simulink model "exercicio3"  (R2018b)
settings: Solver=VariableStepAuto  StartTime=0.0  StopTime=10.0  RelTol=1e-3
values from neighbouring files (symbols this model uses):
  A = [   -1,    1,    2,    2.5 ... (first row only)    [exercicio_01.m]    (also in exercicio_03.m = [-2.068, -2; 2, 0]; exercicio_03_2.m = [-2.068, -2; 2, 0])
  B = [1; 0]    [exercicio_03.m]    (also in exercicio_03_2.m)
  C = [1, -0.4]    [exercicio_03.m]    (also in exercicio_03_2.m)
  D = 0    [exercicio_03.m]    (also in exercicio_03_2.m)
settings Model: Creator=bernardo  LastModifiedBy=bernardo

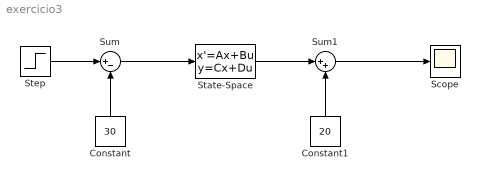
== system exercicio3 ==
  Constant : Constant  Value=30
  Constant1 : Constant  Value=20
  Scope : Scope
  State-Space : StateSpace  A=A  B=B  C=C  D=D  InitialCondition=0.1
  Step : Step  Time=0  After=25  SampleTime=0.001
  Sum : Sum  Inputs=|+-
  Sum1 : Sum  Inputs=|++
  wires:
  Step/1 -> Sum/1
  Sum/1 -> State-Space/1
  Constant/1 -> Sum/2
  State-Space/1 -> Sum1/1
  Constant1/1 -> Sum1/2
  Sum1/1 -> Scope/1
